simulink model "pipeline_blk"  (R2019a)
settings: Solver=VariableStepAuto  StartTime=0.0  StopTime=10.0  RelTol=1e-3
libraries: xbsIndex_r4 x2
settings Model: Creator=mybur  LastModifiedBy=mybur

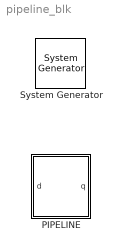
== system pipeline_blk ==
  " System Generator" : xbsIndex_r4/ System Generator  Tag=genX  xilinxfamily=kintex7  part=xc7k325t  speed=-3  package=fbg676  synthesis_tool=Vivado  clock_wrapper=Clock Enables  directory=./netlist  proj_type=Vivado  Synth_file=Vivado Synthesis Defaults  Impl_file=Vivado Implementation Defaults  testbench=off  simulink_period=1  sysclk_period=10  dcm_input_clock_period=10  incr_netlist=off  trim_vbits=Everywhere in SubSystem  dbl_ovrd=According to Block Masks  core_generation=According to Block Masks  run_coregen=off  deprecated_control=off  eval_field=0  block_type=sysgen
  PIPELINE : Subsystem  mask(pipeline){pipeline_len=4}
      mask prompts: pipeline_len "Latency"
      mask help: An explicitly laid-out delay line for use in pipelining to help achieve timing closure.
      mask init:
      | Simulink.Block.eval([gcb, '/pipeline']);

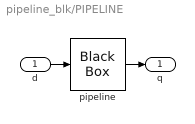
== system pipeline_blk/PIPELINE ==
  d : Inport
  pipeline : xbsIndex_r4/Black Box  init_code=pipeline_config  sim_method=ISE Simulator  verbose=off  block_type=blackbox2
  q : Outport
  wires:
  pipeline/1 -> q/1
  d/1 -> pipeline/1
